simulink model "model_parking_sensorRadar"  (R2022a)
settings: Solver=FixedStepDiscrete  StartTime=0.0  StopTime=2  RelTol=1e-3
model workspace (MAT data in the model file):
  firstWarning = 1
  originalScenarioChecksum = '1DC5E61E13F86F40A5560C8AA035506E'
values from neighbouring files (symbols this model uses):
  Ts = 0.1    [Configuration.m]    (also in test_sim_10000Ep_v10.mat; test_sim_10000Ep_v12_G_oldScen.mat; test_sim_10000Ep_v1_dist.mat; test_sim_1000Ep.mat)
undefined symbols (not defined in the file or in its folder): driving
libraries: drivingscenarioandsensors x8
(part 1 of 2)
settings Model: Creator=User  LastModifiedBy=User

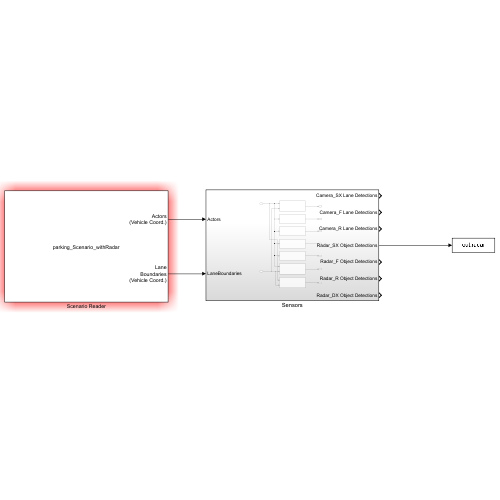
[thumbnail: Simulink's stored preview of the top-level diagram]
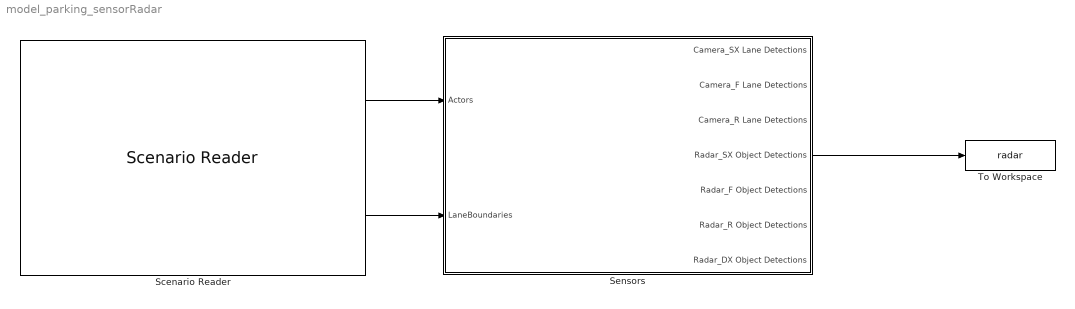
== system model_parking_sensorRadar ==
  Scenario Reader : drivingscenarioandsensors/Scenario Reader  ScenarioSource=From file  ScenarioFileName=C:\Users\User\OneDrive\Desktop\Thesis_Project\project\parking_Scenario_withRadar.mat  ScenarioVariableName=scenario  OutputCoordinateSystem=Vehicle coordinates  EgoVehicleSource=Scenario  EgoVehicleActorID=1  OrientVehiclesOnRoad=off  OutputEgoVehiclePose=off  OutputEgoVehicleState=off  SampleTime=Ts  LaneBoundaryOutput=Ego vehicle lane boundaries  LaneBoundaryDistance=linspace(-150, 150, 101)  LaneBoundaryLocation=Center of lane markings  BusNameSource=Auto  BusName=BusActors  BusNumActorsSource=Scenario  BusNumActors=100  BusName2Source=Auto  BusName2=BusLaneBoundaries  BusNumLaneBoundariesSource=Scenario  BusNumLaneBoundaries=10  BusName3Source=Auto  BusName3=BusEgoActor  BusName4Source=Auto  BusName4=BusEgoState  ShowCoordinateLabels=on  SimulateUsing=Interpreted execution
  Sensors : Subsystem
  To Workspace : ToWorkspace  VariableName=radar  SaveFormat=Timeseries  SampleTime=-1
  wires:
  Scenario Reader/1 -> Sensors/1(Actors)
  Scenario Reader/2 -> Sensors/2(LaneBoundaries)
  Sensors/4(Radar_SX Object Detections) -> To Workspace/1
